simulink model "Latex"  (R2023a)
settings: Solver=VariableStepAuto  StartTime=0.0  StopTime=10.0  RelTol=1e-3
undefined symbols (not defined in the file): A, A_motor, B, B_mag0, B_motor, C_motor, D_motor, I, J, K3_2, K_gamma, Ke, Kt, La, n_cal, R_mgt, Ra, RW_omega_max, T_ext, T_max, T_max_mgt
libraries: matrix_library x5, slpidlib x2, vrlib x1
settings Model: Creator=Personal  LastModifiedBy=Personal

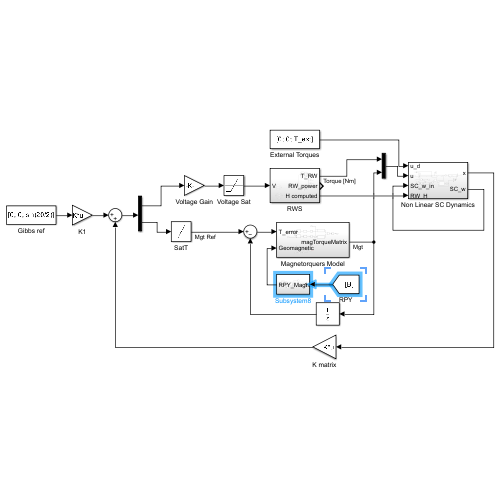
[thumbnail: Simulink's stored preview of the top-level diagram]
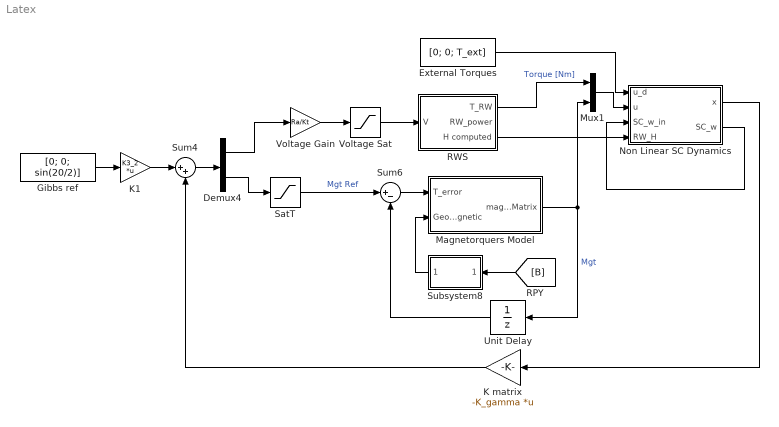
== system Latex ==
  Demux4 : Demux  Outputs=2
  External Torques : Constant  Value=[0; 0; T_ext]
  Gibbs ref : Constant  Value=[0; 0; sin(20/2)]
  K matrix : Gain  Gain=-K_gamma  Multiplication=Matrix(K*u)
  K1 : Gain  Gain=K3_2  Multiplication=Matrix(K*u)
  Magnetorquers Model : Subsystem
  Mux1 : Mux  Inputs=2
  Non Linear SC Dynamics : Subsystem
  RWS : Subsystem
  SatT : Saturate  UpperLimit=T_max_mgt  LowerLimit=-T_max_mgt
  Subsystem8 : Subsystem
  Sum4 : Sum  Inputs=|++
  Sum6 : Sum  Inputs=|+-
  Unit Delay : UnitDelay  SampleTime=-1  HasFrameUpgradeWarning=on
  Voltage Gain : Gain  Gain=Ra/Kt
  Voltage Sat : Saturate  UpperLimit=6  LowerLimit=-6
  wires:
  RWS/3(H computed) -> Non Linear SC Dynamics/4(RW_H)
  Magnetorquers Model/1(magTorqueMatrix) -> Mux1/2, Unit Delay/1  "Mgt"
  SatT/1 -> Sum6/1  "Mgt Ref"
  Non Linear SC Dynamics/2(SC_w) -> Non Linear SC Dynamics/3(SC_w_in)
  [B] -> Subsystem8/1(Input)
  K matrix/1 -> Sum4/2
  Demux4/2 -> SatT/1
  Demux4/1 -> Voltage Gain/1
  Voltage Gain/1 -> Voltage Sat/1
  Sum6/1 -> Magnetorquers Model/1(T_error)
  External Torques/1 -> Non Linear SC Dynamics/1(u_d)
  Voltage Sat/1 -> RWS/1(V)
  K1/1 -> Sum4/1
  Non Linear SC Dynamics/1(x) -> K matrix/1
  RWS/1(T_RW) -> Mux1/1  "Torque [Nm]"
  Mux1/1 -> Non Linear SC Dynamics/2(u)
  Unit Delay/1 -> Sum6/2
  Sum4/1 -> Demux4/1
  Subsystem8/1(RPY_Magnetic) -> Magnetorquers Model/2(Geomagnetic)
  Gibbs ref/1 -> K1/1

== system Latex/Magnetorquers Model ==
  T_error : Inport
  Geomagnetic : Inport  Port=2
  Add : Sum
  Add2 : Sum  Commented=on
  Corrección X : MATLAB Function  TreatAsAtomicUnit=on
  Corrección Y : MATLAB Function  TreatAsAtomicUnit=on
  Demux : Demux  Outputs=3
  From : From  Commented=on  GotoTag=V1
  From1 : From  Commented=on  GotoTag=V2
  Gain : Gain  Commented=on  Gain=1/R_mgt
  Gain1 : Gain  Commented=on  Gain=1/R_mgt
  Geomagnetic1 : InportShadow  Port=2
  Mgt X : Subsystem
  Mgt Y : Subsystem
  PID Controller1 : slpidlib/PID Controller  Controller=PID  Form=Parallel  TimeDomain=Continuous-time  UseExternalTs=off  SampleTime=-1  IntegratorMethod=Forward Euler  FilterMethod=Forward Euler  ControllerParametersSource=internal  P=0  I=2538362.26384975  UseKiTs=off  D=0  N=100  UseFilter=on  TunerSelectOption=Transfer Function Based (PID Tuner App)  InitialConditionSource=internal  InitialConditionForIntegrator=0  InitialConditionForFilter=0  DifferentiatorICPrevScaledInput=0  ExternalReset=none  TrackingMode=off  Kt=1  LimitOutput=on  SatLimitsSource=internal  UpperSaturationLimit=5  LowerSaturationLimit=-5  LinearizeAsGain=on  AntiWindupMode=clamping  Kb=1  LimitIntegrator=off  UpperIntegratorSaturationLimit=inf  LowerIntegratorSaturationLimit=-inf  POutMin=[]  POutMax=[]  IOutMin=[]  IOutMax=[]  DOutMin=[]  DOutMax=[]  NOutMin=[]  NOutMax=[]  SumOutMin=[]  SumOutMax=[]  SaturationOutMin=[]  SaturationOutMax=[]  PParamMin=[]  PParamMax=[]  IParamMin=[]  IParamMax=[]  DParamMin=[]  DParamMax=[]  NParamMin=[]  NParamMax=[]  KbParamMin=[]  KbParamMax=[]  KtParamMin=[]  KtParamMax=[]  KbOutMin=[]  KbOutMax=[]  KtOutMin=[]  KtOutMax=[]  IntegratorOutMin=[]  IntegratorOutMax=[]  FilterOutMin=[]  FilterOutMax=[]  SumI1OutMin=[]  SumI1OutMax=[]  SumI2OutMin=[]  SumI2OutMax=[]  SumI3OutMin=[]  SumI3OutMax=[]  SumI4OutMin=[]  SumI4OutMax=[]  SumDOutMin=[]  SumDOutMax=[]  DifferentiatorOutMin=[]  DifferentiatorOutMax=[]  FilterDiffOutCoefMin=[]  FilterDiffOutCoefMax=[]  ReciprocalOutMin=[]  ReciprocalOutMax=[]  SumDenOutMin=[]  SumDenOutMax=[]  SumNumOutMin=[]  SumNumOutMax=[]  DivideOutMin=[]  DivideOutMax=[]  UdiffTsProdOutMin=[]  UdiffTsProdOutMax=[]  NTsProdOutMin=[]  NTsProdOutMax=[]  UintegralTsProdOutMin=[]  UintegralTsProdOutMax=[]  UngainTsProdOutMin=[]  UngainTsProdOutMax=[]  ClampingZeroOutDataTypeStr=Inherit: Inherit via back propagation  ClampingZeroOutMin=[]  ClampingZeroOutMax=[]  FilterDenConstantOutDataTypeStr=Inherit: Inherit via back propagation  FilterDenConstantOutMin=[]  FilterDenConstantOutMax=[]  PCopyOutDataTypeStr=Inherit: Inherit via back propagation  PCopyOutMin=[]  PCopyOutMax=[]  NCopyOutDataTypeStr=Inherit: Inherit via back propagation  NCopyOutMin=[]  NCopyOutMax=[]  IntegratorContinuousStateAttributes=''  IntegratorStateMustResolveToSignalObject=off  IntegratorRTWStateStorageClass=Auto  FilterContinuousStateAttributes=''  FilterStateMustResolveToSignalObject=off  FilterRTWStateStorageClass=Auto  ParallelPVariant=InternalParameters  IdealPVariant=Disabled  IVariant=InternalParameters  DVariant=InternalParameters  IntegratorVariant=Continuous  SatVariant=Enabled  AWVariant=ContClampingParallel  PCopyVariant=Disabled  TRVariant=Disabled  FdbkBlocksVariant=Forward  IdealPFdbkVariant=Disabled  SatFdbkVariant=Disabled  DerivativeFilterVariant=ContFilter  NVariant=InternalParameters  NCopyVariant=Disabled  FilterICVariant=InternalICsFilter  IntegratorICVariant=InternalICs  ExternalResetVariant=Disabled  TRSumVariant=Passthrough  SumFdbkVariant=Disabled  SumVariant=Sum_PID  TsampFilterVariant=InternalTs  TsampNgainVariant=Passthrough  TsampIntegralVariant=Disabled_SignalSpec  ExternalSaturationOutDataTypeStr=Inherit: Same as second input
  PID Controller5 : slpidlib/PID Controller  Controller=PID  Form=Parallel  TimeDomain=Continuous-time  UseExternalTs=off  SampleTime=-1  IntegratorMethod=Forward Euler  FilterMethod=Forward Euler  ControllerParametersSource=internal  P=0  I=2538362.26384975  UseKiTs=off  D=0  N=100  UseFilter=on  TunerSelectOption=Transfer Function Based (PID Tuner App)  InitialConditionSource=internal  InitialConditionForIntegrator=0  InitialConditionForFilter=0  DifferentiatorICPrevScaledInput=0  ExternalReset=none  TrackingMode=off  Kt=1  LimitOutput=on  SatLimitsSource=internal  UpperSaturationLimit=5  LowerSaturationLimit=-5  LinearizeAsGain=on  AntiWindupMode=clamping  Kb=1  LimitIntegrator=off  UpperIntegratorSaturationLimit=inf  LowerIntegratorSaturationLimit=-inf  POutMin=[]  POutMax=[]  IOutMin=[]  IOutMax=[]  DOutMin=[]  DOutMax=[]  NOutMin=[]  NOutMax=[]  SumOutMin=[]  SumOutMax=[]  SaturationOutMin=[]  SaturationOutMax=[]  PParamMin=[]  PParamMax=[]  IParamMin=[]  IParamMax=[]  DParamMin=[]  DParamMax=[]  NParamMin=[]  NParamMax=[]  KbParamMin=[]  KbParamMax=[]  KtParamMin=[]  KtParamMax=[]  KbOutMin=[]  KbOutMax=[]  KtOutMin=[]  KtOutMax=[]  IntegratorOutMin=[]  IntegratorOutMax=[]  FilterOutMin=[]  FilterOutMax=[]  SumI1OutMin=[]  SumI1OutMax=[]  SumI2OutMin=[]  SumI2OutMax=[]  SumI3OutMin=[]  SumI3OutMax=[]  SumI4OutMin=[]  SumI4OutMax=[]  SumDOutMin=[]  SumDOutMax=[]  DifferentiatorOutMin=[]  DifferentiatorOutMax=[]  FilterDiffOutCoefMin=[]  FilterDiffOutCoefMax=[]  ReciprocalOutMin=[]  ReciprocalOutMax=[]  SumDenOutMin=[]  SumDenOutMax=[]  SumNumOutMin=[]  SumNumOutMax=[]  DivideOutMin=[]  DivideOutMax=[]  UdiffTsProdOutMin=[]  UdiffTsProdOutMax=[]  NTsProdOutMin=[]  NTsProdOutMax=[]  UintegralTsProdOutMin=[]  UintegralTsProdOutMax=[]  UngainTsProdOutMin=[]  UngainTsProdOutMax=[]  ClampingZeroOutDataTypeStr=Inherit: Inherit via back propagation  ClampingZeroOutMin=[]  ClampingZeroOutMax=[]  FilterDenConstantOutDataTypeStr=Inherit: Inherit via back propagation  FilterDenConstantOutMin=[]  FilterDenConstantOutMax=[]  PCopyOutDataTypeStr=Inherit: Inherit via back propagation  PCopyOutMin=[]  PCopyOutMax=[]  NCopyOutDataTypeStr=Inherit: Inherit via back propagation  NCopyOutMin=[]  NCopyOutMax=[]  IntegratorContinuousStateAttributes=''  IntegratorStateMustResolveToSignalObject=off  IntegratorRTWStateStorageClass=Auto  FilterContinuousStateAttributes=''  FilterStateMustResolveToSignalObject=off  FilterRTWStateStorageClass=Auto  ParallelPVariant=InternalParameters  IdealPVariant=Disabled  IVariant=InternalParameters  DVariant=InternalParameters  IntegratorVariant=Continuous  SatVariant=Enabled  AWVariant=ContClampingParallel  PCopyVariant=Disabled  TRVariant=Disabled  FdbkBlocksVariant=Forward  IdealPFdbkVariant=Disabled  SatFdbkVariant=Disabled  DerivativeFilterVariant=ContFilter  NVariant=InternalParameters  NCopyVariant=Disabled  FilterICVariant=InternalICsFilter  IntegratorICVariant=InternalICs  ExternalResetVariant=Disabled  TRSumVariant=Passthrough  SumFdbkVariant=Disabled  SumVariant=Sum_PID  TsampFilterVariant=InternalTs  TsampNgainVariant=Passthrough  TsampIntegralVariant=Disabled_SignalSpec  ExternalSaturationOutDataTypeStr=Inherit: Same as second input
  SatT3 : Saturate  UpperLimit=T_max_mgt  LowerLimit=-T_max_mgt
  Saturation 6V1 : Saturate  UpperLimit=5  LowerLimit=-5
  Saturation 6V2 : Saturate  UpperLimit=5  LowerLimit=-5
  Square : Math  Commented=on  Operator=square
  Square1 : Math  Commented=on  Operator=square
  magTorqueMatrix : Outport
  wires:
  Saturation 6V1/1 -> Mgt X/2(PWR)  "PWR_mgt X"
  PID Controller1/1 -> Saturation 6V2/1
  PID Controller5/1 -> Saturation 6V1/1
  Saturation 6V2/1 -> Mgt Y/2(PWR)  "PWR_mgt Y"
  Add/1 -> SatT3/1
  T_error/1 -> Demux/1
  Mgt X/1(Mgt XYZ) -> Add/1
  Mgt Y/1(Mgt XYZ) -> Add/2
  Demux/3 -> Corrección X/1("T_error "), Corrección Y/1("T_error ")
  Corrección X/1(T_error) -> PID Controller5/1
  Geomagnetic1/1 -> Corrección X/2(B), Corrección Y/2(B)
  Corrección Y/1(T_error) -> PID Controller1/1
  Square1/1 -> Gain1/1
  From/1 -> Square/1
  Gain1/1 -> Add2/2
  Square/1 -> Gain/1
  Gain/1 -> Add2/1
  Add2/1 -> ?
  From1/1 -> Square1/1
  Geomagnetic/1 -> Mgt Y/1(B), Mgt X/1(B)
  SatT3/1 -> magTorqueMatrix/1  "Mgt"

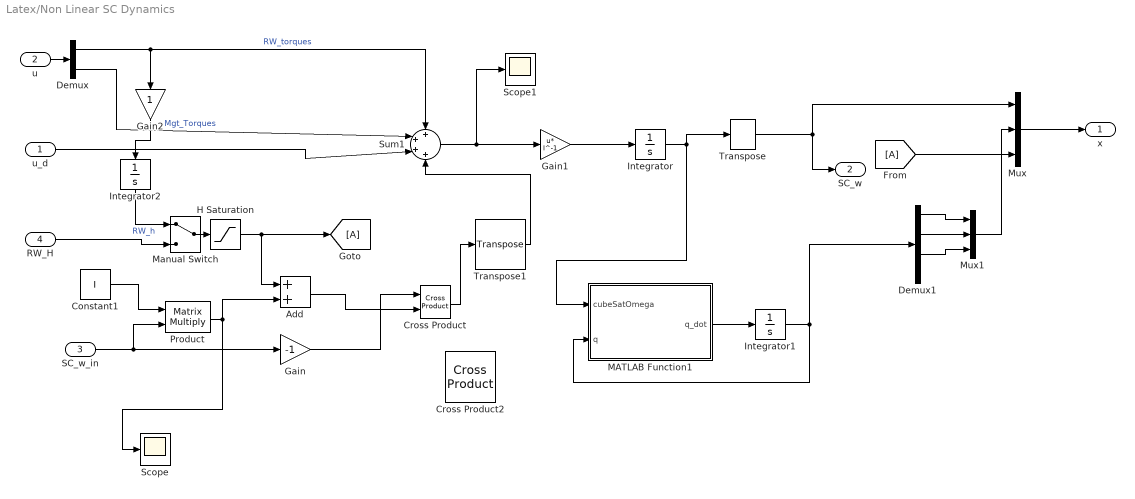
== system Latex/Non Linear SC Dynamics ==
  u_d : Inport
  u : Inport  Port=2
  SC_w_in : Inport  Port=3
  RW_H : Inport  Port=4
  Add : Sum
  Constant1 : Constant  Value=I
  Cross Product : vrlib/Utilities/Cross Product
  Cross Product2 : matrix_library/Cross Product
  Demux : Demux  Outputs=2
  Demux1 : Demux
  From : From
  Gain : Gain  Gain=-1
  Gain1 : Gain  Gain=I^-1  Multiplication=Matrix(u*K)
  Gain2 : Gain
  Goto : Goto
  H Saturation : Saturate  UpperLimit=J*RW_omega_max  LowerLimit=-J*RW_omega_max
  Integrator : Integrator  InitialCondition=[0 0 0]
  Integrator1 : Integrator  InitialCondition=[0 0 0 1]
  Integrator2 : Integrator  InitialCondition=[0 0 0]
  MATLAB Function1 : MATLAB Function  TreatAsAtomicUnit=on
  Manual Switch : ManualSwitch
  Mux : Mux  Inputs=3
  Mux1 : Mux  Inputs=3
  Product : Product  Multiplication=Matrix(*)
  Scope : Scope
  Scope1 : Scope
  Sum1 : Sum  Inputs=++++
  Transpose : matrix_library/Transpose
  Transpose1 : matrix_library/Transpose
  x : Outport
  SC_w : Outport  Port=2
  wires:
  Demux/1 -> Sum1/1, Gain2/1  "RW_torques"
  u_d/1 -> Sum1/3
  Integrator1/1 -> Demux1/1, MATLAB Function1/2(q)
  Constant1/1 -> Product/1
  Product/1 -> Scope/1, Add/2
  Gain/1 -> Cross Product/1
  Add/1 -> Cross Product/2
  Cross Product/1 -> Transpose1/1
  Sum1/1 -> Scope1/1, Gain1/1
  Gain1/1 -> Integrator/1
  Integrator/1 -> MATLAB Function1/1(cubeSatOmega), Transpose/1
  MATLAB Function1/1(q_dot) -> Integrator1/1
  SC_w_in/1 -> Product/2, Gain/1
  Transpose/1 -> SC_w/1, Mux/1
  Transpose1/1 -> Sum1/4
  Demux/2 -> Sum1/2  "Mgt_Torques"
  u/1 -> Demux/1
  Mux/1 -> x/1
  Demux1/1 -> Mux1/1
  Demux1/2 -> Mux1/2
  Demux1/3 -> Mux1/3
  Mux1/1 -> Mux/2
  From/1 -> Mux/3
  H Saturation/1 -> Goto/1, Add/1
  RW_H/1 -> Manual Switch/2
  Manual Switch/1 -> H Saturation/1
  Integrator2/1 -> Manual Switch/1  "RW_h"
  Gain2/1 -> Integrator2/1

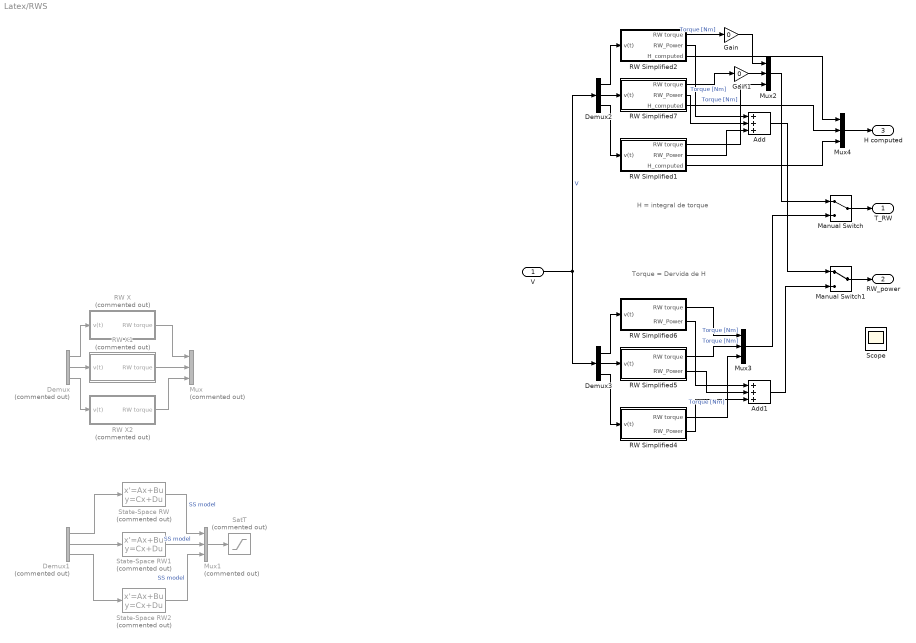
== system Latex/RWS ==
  note: Torque = Dervida de H
  note: H = integral de torque
  V : Inport
  Add : Sum  Inputs=+++
  Add1 : Sum  Inputs=+++
  Demux : Demux  Commented=on  Outputs=3
  Demux1 : Demux  Commented=on  Outputs=3
  Demux2 : Demux  Outputs=3
  Demux3 : Demux  Outputs=3
  Gain : Gain  Gain=0
  Gain1 : Gain  Gain=0
  Manual Switch : ManualSwitch
  Manual Switch1 : ManualSwitch
  Mux : Mux  Commented=on  Inputs=3
  Mux1 : Mux  Commented=on  Inputs=3
  Mux2 : Mux  Inputs=3
  Mux3 : Mux  Inputs=3
  Mux4 : Mux  Inputs=3
  RW Simplified1 : Subsystem
  RW Simplified2 : Subsystem
  RW Simplified4 : Subsystem
  RW Simplified5 : Subsystem
  RW Simplified6 : Subsystem
  RW Simplified7 : Subsystem
  RW X : Subsystem  Commented=on
  RW X1 : Subsystem  Commented=on
  RW X2 : Subsystem  Commented=on
  SatT : Saturate  Commented=on  UpperLimit=T_max  LowerLimit=-T_max
  Scope : Scope
  State-Space RW : StateSpace  Commented=on  A=A_motor  B=B_motor  C=C_motor  D=D_motor  InitialCondition=0
  State-Space RW1 : StateSpace  Commented=on  A=A_motor  B=B_motor  C=C_motor  D=D_motor  InitialCondition=0
  State-Space RW2 : StateSpace  Commented=on  A=A_motor  B=B_motor  C=C_motor  D=D_motor  InitialCondition=0
  T_RW : Outport
  RW_power : Outport  Port=2
  H computed : Outport  Port=3
  wires:
  Demux/1 -> RW X/1(v(t))
  V/1 -> Demux2/1, Demux3/1  "V"
  Demux/3 -> RW X2/1(v(t))
  Demux/2 -> RW X1/1(v(t))
  RW X2/1(RW torque) -> Mux/3
  Demux1/1 -> State-Space RW/1
  Demux1/2 -> State-Space RW1/1
  Demux1/3 -> State-Space RW2/1
  State-Space RW1/1 -> Mux1/2  "SS model"
  State-Space RW/1 -> Mux1/1  "SS model"
  State-Space RW2/1 -> Mux1/3  "SS model"
  Mux1/1 -> SatT/1
  RW Simplified1/2(RW_Power) -> Add/3
  Manual Switch/1 -> T_RW/1
  RW X/1(RW torque) -> Mux/1
  RW X1/1(RW torque) -> Mux/2
  Demux2/1 -> RW Simplified2/1(v(t))
  Demux2/2 -> RW Simplified7/1(v(t))
  Demux2/3 -> RW Simplified1/1(v(t))
  RW Simplified2/1(RW torque) -> Gain/1  "Torque [Nm]"
  RW Simplified7/1(RW torque) -> Gain1/1  "Torque [Nm]"
  RW Simplified1/1(RW torque) -> Mux2/3  "Torque [Nm]"
  Mux2/1 -> Manual Switch/1
  RW Simplified7/2(RW_Power) -> Add/2
  RW Simplified2/2(RW_Power) -> Add/1
  Add/1 -> Manual Switch1/1
  RW Simplified6/2(RW_Power) -> Add1/1
  RW Simplified5/2(RW_Power) -> Add1/2
  Mux3/1 -> Manual Switch/2
  RW Simplified4/1(RW torque) -> Mux3/3  "Torque [Nm]"
  RW Simplified5/1(RW torque) -> Mux3/2  "Torque [Nm]"
  RW Simplified6/1(RW torque) -> Mux3/1  "Torque [Nm]"
  Demux3/3 -> RW Simplified4/1(v(t))
  Demux3/2 -> RW Simplified5/1(v(t))
  Demux3/1 -> RW Simplified6/1(v(t))
  RW Simplified4/2(RW_Power) -> Add1/3
  Add1/1 -> Manual Switch1/2
  Manual Switch1/1 -> RW_power/1
  RW Simplified1/3(H_computed) -> Mux4/3
  RW Simplified2/3(H_computed) -> Mux4/1
  RW Simplified7/3(H_computed) -> Mux4/2
  Mux4/1 -> H computed/1
  Gain/1 -> Mux2/1
  Gain1/1 -> Mux2/2

== system Latex/Subsystem8 ==
  Input : Inport
  Clock : Clock
  Constant1 : Constant  Value=B_mag0
  Extract B : MATLAB Function  TreatAsAtomicUnit=on
  MATLAB Function : MATLAB Function  TreatAsAtomicUnit=on
  Scope1 : Scope
  Scope8 : Scope
  Zero-Order Hold : ZeroOrderHold  SampleTime=-1
  RPY_Magnetic : Outport
  wires:
  Constant1/1 -> Extract B/1(B_cal)
  Extract B/1(XYZ_Magnetic) -> MATLAB Function/1(NEDMagnetic), Scope8/1
  Input/1 -> MATLAB Function/2(RPY)
  Zero-Order Hold/1 -> Scope1/1, Extract B/2(time)
  MATLAB Function/1(RPY_Magnetic) -> RPY_Magnetic/1
  Clock/1 -> Zero-Order Hold/1

== system Latex/Magnetorquers Model/Mgt X ==
  B : Inport
  PWR : Inport  Port=2
  Cross Product : matrix_library/Cross Product
  Mgt_ejeX : Gain  Gain=[1 0 0]
  "Momento Dipolar " : Gain  Gain=n_cal*A/R_mgt
  Mgt XYZ : Outport
  wires:
  "Momento Dipolar "/1 -> Mgt_ejeX/1
  Mgt_ejeX/1 -> Cross Product/1
  Cross Product/1 -> Mgt XYZ/1  "MgtX"
  PWR/1 -> "Momento Dipolar "/1
  B/1 -> Cross Product/2

== system Latex/Magnetorquers Model/Mgt Y ==
  B : Inport
  PWR : Inport  Port=2
  Cross Product : matrix_library/Cross Product
  Mgt_ejeY : Gain  Gain=[0 1 0]
  "Momento Dipolar " : Gain  Gain=n_cal*A/R_mgt
  Mgt XYZ : Outport
  wires:
  B/1 -> Cross Product/2
  PWR/1 -> "Momento Dipolar "/1
  Cross Product/1 -> Mgt XYZ/1  "MgtX"
  Mgt_ejeY/1 -> Cross Product/1
  "Momento Dipolar "/1 -> Mgt_ejeY/1

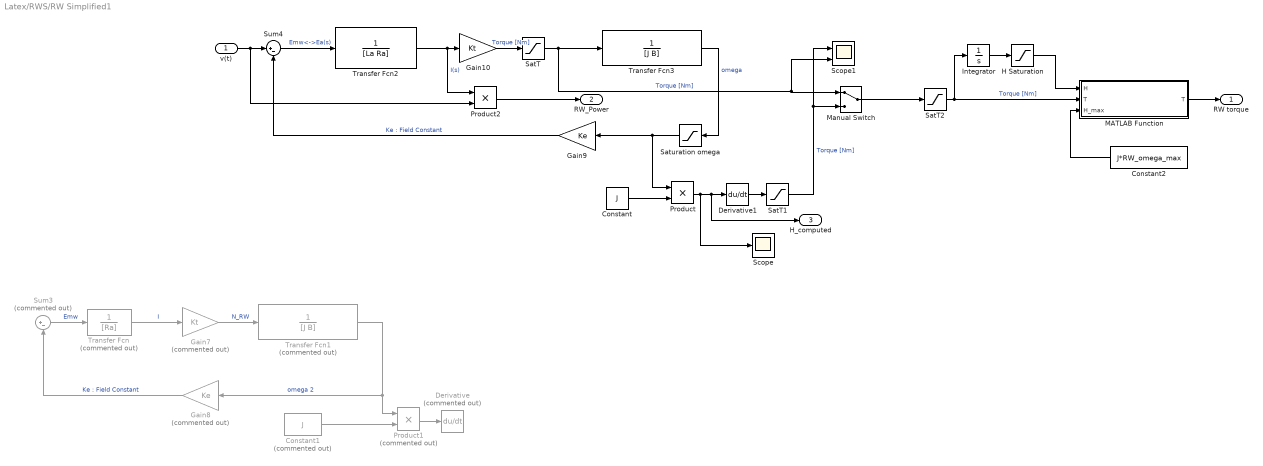
== system Latex/RWS/RW Simplified1 ==
  v(t) : Inport
  Constant : Constant  Value=J
  Constant1 : Constant  Commented=on  Value=J
  Constant2 : Constant  Value=J*RW_omega_max
  Derivative : Derivative  Commented=on
  Derivative1 : Derivative
  Gain10 : Gain  Gain=Kt
  Gain7 : Gain  Commented=on  Gain=Kt
  Gain8 : Gain  Commented=on  Gain=Ke
  Gain9 : Gain  Gain=Ke
  H Saturation : Saturate  UpperLimit=J*RW_omega_max  LowerLimit=-J*RW_omega_max
  Integrator : Integrator
  MATLAB Function : MATLAB Function  TreatAsAtomicUnit=on
  Manual Switch : ManualSwitch
  Product : Product
  Product1 : Product  Commented=on
  Product2 : Product
  SatT : Saturate  UpperLimit=T_max  LowerLimit=-T_max
  SatT1 : Saturate  UpperLimit=T_max  LowerLimit=-T_max
  SatT2 : Saturate  UpperLimit=T_max  LowerLimit=-T_max
  Saturation omega : Saturate  UpperLimit=RW_omega_max  LowerLimit=-RW_omega_max
  Scope : Scope
  Scope1 : Scope  NumInputPorts=2
  Sum3 : Sum  Commented=on  Inputs=|+-
  Sum4 : Sum  Inputs=|+-
  Transfer Fcn : TransferFcn  Commented=on  Denominator=[Ra]
  Transfer Fcn1 : TransferFcn  Commented=on  Denominator=[J B]
  Transfer Fcn2 : TransferFcn  Denominator=[La Ra]
  Transfer Fcn3 : TransferFcn  Denominator=[J B]
  RW torque : Outport  VectorParamsAs1DForOutWhenUnconnected=off
  RW_Power : Outport  Port=2  VectorParamsAs1DForOutWhenUnconnected=off
  H_computed : Outport  Port=3
  wires:
  Transfer Fcn2/1 -> Product2/1, Gain10/1  "I(s)"
  Sum4/1 -> Transfer Fcn2/1  "Emw<->Ea(s)"
  Gain9/1 -> Sum4/2  "Ke : Field Constant"
  Transfer Fcn3/1 -> Saturation omega/1  "omega"
  Constant/1 -> Product/2
  v(t)/1 -> Product2/2, Sum4/1
  Product1/1 -> Derivative/1
  Constant1/1 -> Product1/2
  Transfer Fcn1/1 -> Product1/1, Gain8/1  "omega 2"
  Gain7/1 -> Transfer Fcn1/1  "N_RW"
  Sum3/1 -> Transfer Fcn/1  "Emw"
  Transfer Fcn/1 -> Gain7/1  "I"
  Gain8/1 -> Sum3/2  "Ke : Field Constant"
  Gain10/1 -> SatT/1  "Torque [Nm]"
  SatT/1 -> Manual Switch/1, Scope1/2, Transfer Fcn3/1  "Torque [Nm]"
  Product2/1 -> RW_Power/1
  Product/1 -> Scope/1, H_computed/1, Derivative1/1
  Derivative1/1 -> SatT1/1
  SatT1/1 -> Scope1/1, Manual Switch/2  "Torque [Nm]"
  Manual Switch/1 -> SatT2/1
  Saturation omega/1 -> Product/1, Gain9/1
  SatT2/1 -> MATLAB Function/2("T "), Integrator/1  "Torque [Nm]"
  Integrator/1 -> H Saturation/1
  Constant2/1 -> MATLAB Function/3(H_max)
  H Saturation/1 -> MATLAB Function/1(H)
  MATLAB Function/1(T) -> RW torque/1

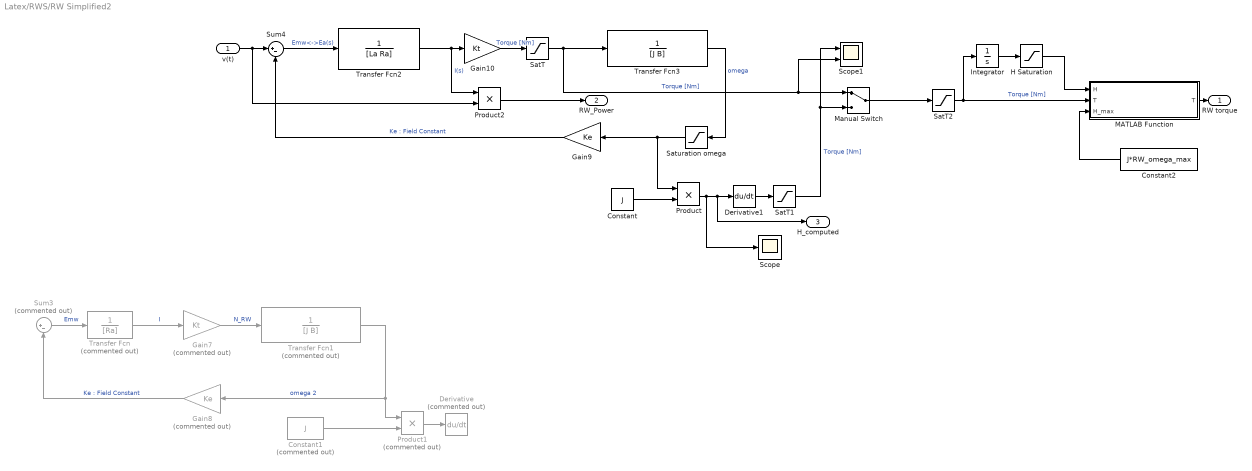
== system Latex/RWS/RW Simplified2 ==
  v(t) : Inport
  Constant : Constant  Value=J
  Constant1 : Constant  Commented=on  Value=J
  Constant2 : Constant  Value=J*RW_omega_max
  Derivative : Derivative  Commented=on
  Derivative1 : Derivative
  Gain10 : Gain  Gain=Kt
  Gain7 : Gain  Commented=on  Gain=Kt
  Gain8 : Gain  Commented=on  Gain=Ke
  Gain9 : Gain  Gain=Ke
  H Saturation : Saturate  UpperLimit=J*RW_omega_max  LowerLimit=-J*RW_omega_max
  Integrator : Integrator
  MATLAB Function : MATLAB Function  TreatAsAtomicUnit=on
  Manual Switch : ManualSwitch
  Product : Product
  Product1 : Product  Commented=on
  Product2 : Product
  SatT : Saturate  UpperLimit=T_max  LowerLimit=-T_max
  SatT1 : Saturate  UpperLimit=T_max  LowerLimit=-T_max
  SatT2 : Saturate  UpperLimit=T_max  LowerLimit=-T_max
  Saturation omega : Saturate  UpperLimit=RW_omega_max  LowerLimit=-RW_omega_max
  Scope : Scope
  Scope1 : Scope  NumInputPorts=2
  Sum3 : Sum  Commented=on  Inputs=|+-
  Sum4 : Sum  Inputs=|+-
  Transfer Fcn : TransferFcn  Commented=on  Denominator=[Ra]
  Transfer Fcn1 : TransferFcn  Commented=on  Denominator=[J B]
  Transfer Fcn2 : TransferFcn  Denominator=[La Ra]
  Transfer Fcn3 : TransferFcn  Denominator=[J B]
  RW torque : Outport  VectorParamsAs1DForOutWhenUnconnected=off
  RW_Power : Outport  Port=2  VectorParamsAs1DForOutWhenUnconnected=off
  H_computed : Outport  Port=3
  wires:
  Transfer Fcn2/1 -> Product2/1, Gain10/1  "I(s)"
  Sum4/1 -> Transfer Fcn2/1  "Emw<->Ea(s)"
  Gain9/1 -> Sum4/2  "Ke : Field Constant"
  Transfer Fcn3/1 -> Saturation omega/1  "omega"
  Constant/1 -> Product/2
  v(t)/1 -> Product2/2, Sum4/1
  Product1/1 -> Derivative/1
  Constant1/1 -> Product1/2
  Transfer Fcn1/1 -> Product1/1, Gain8/1  "omega 2"
  Gain7/1 -> Transfer Fcn1/1  "N_RW"
  Sum3/1 -> Transfer Fcn/1  "Emw"
  Transfer Fcn/1 -> Gain7/1  "I"
  Gain8/1 -> Sum3/2  "Ke : Field Constant"
  Gain10/1 -> SatT/1  "Torque [Nm]"
  SatT/1 -> Manual Switch/1, Scope1/2, Transfer Fcn3/1  "Torque [Nm]"
  Product2/1 -> RW_Power/1
  Product/1 -> Scope/1, H_computed/1, Derivative1/1
  Derivative1/1 -> SatT1/1
  SatT1/1 -> Scope1/1, Manual Switch/2  "Torque [Nm]"
  Manual Switch/1 -> SatT2/1
  Saturation omega/1 -> Product/1, Gain9/1
  SatT2/1 -> Integrator/1, MATLAB Function/2("T ")  "Torque [Nm]"
  Integrator/1 -> H Saturation/1
  Constant2/1 -> MATLAB Function/3(H_max)
  H Saturation/1 -> MATLAB Function/1(H)
  MATLAB Function/1(T) -> RW torque/1

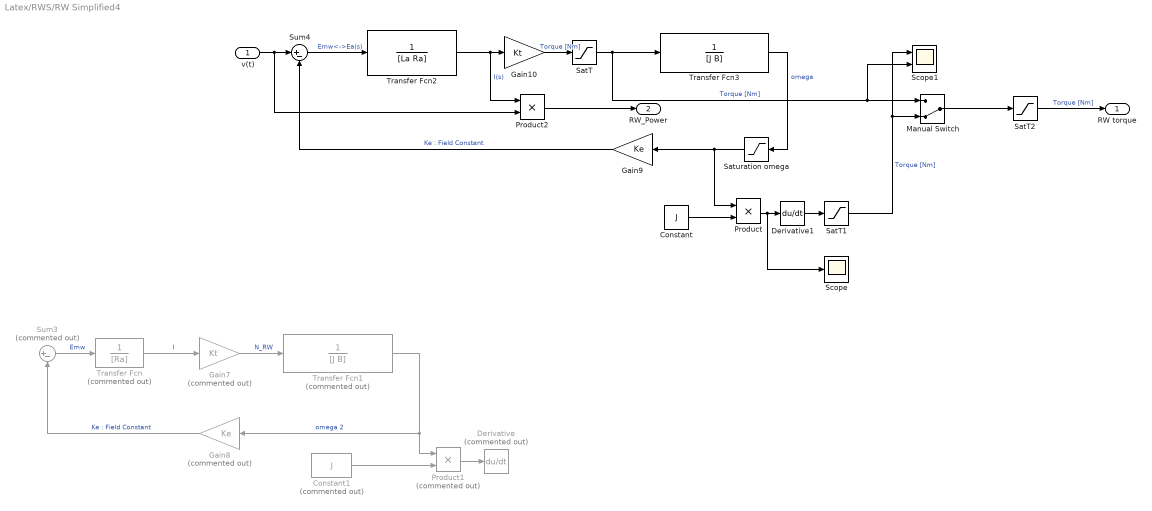
== system Latex/RWS/RW Simplified4 ==
  v(t) : Inport
  Constant : Constant  Value=J
  Constant1 : Constant  Commented=on  Value=J
  Derivative : Derivative  Commented=on
  Derivative1 : Derivative
  Gain10 : Gain  Gain=Kt
  Gain7 : Gain  Commented=on  Gain=Kt
  Gain8 : Gain  Commented=on  Gain=Ke
  Gain9 : Gain  Gain=Ke
  Manual Switch : ManualSwitch  CurrentSetting=0
  Product : Product
  Product1 : Product  Commented=on
  Product2 : Product
  SatT : Saturate  UpperLimit=T_max  LowerLimit=-T_max
  SatT1 : Saturate  UpperLimit=T_max  LowerLimit=-T_max
  SatT2 : Saturate  UpperLimit=T_max  LowerLimit=-T_max
  Saturation omega : Saturate  UpperLimit=RW_omega_max  LowerLimit=-RW_omega_max
  Scope : Scope
  Scope1 : Scope  NumInputPorts=2
  Sum3 : Sum  Commented=on  Inputs=|+-
  Sum4 : Sum  Inputs=|+-
  Transfer Fcn : TransferFcn  Commented=on  Denominator=[Ra]
  Transfer Fcn1 : TransferFcn  Commented=on  Denominator=[J B]
  Transfer Fcn2 : TransferFcn  Denominator=[La Ra]
  Transfer Fcn3 : TransferFcn  Denominator=[J B]
  RW torque : Outport  VectorParamsAs1DForOutWhenUnconnected=off
  RW_Power : Outport  Port=2  VectorParamsAs1DForOutWhenUnconnected=off
  wires:
  SatT2/1 -> RW torque/1  "Torque [Nm]"
  Saturation omega/1 -> Gain9/1, Product/1
  Manual Switch/1 -> SatT2/1
  SatT1/1 -> Manual Switch/2, Scope1/1  "Torque [Nm]"
  Derivative1/1 -> SatT1/1
  Product/1 -> Derivative1/1, Scope/1
  Product2/1 -> RW_Power/1
  SatT/1 -> Transfer Fcn3/1, Scope1/2, Manual Switch/1  "Torque [Nm]"
  Gain10/1 -> SatT/1  "Torque [Nm]"
  Gain8/1 -> Sum3/2  "Ke : Field Constant"
  Transfer Fcn/1 -> Gain7/1  "I"
  Sum3/1 -> Transfer Fcn/1  "Emw"
  Gain7/1 -> Transfer Fcn1/1  "N_RW"
  Transfer Fcn1/1 -> Gain8/1, Product1/1  "omega 2"
  Constant1/1 -> Product1/2
  Product1/1 -> Derivative/1
  v(t)/1 -> Sum4/1, Product2/2
  Constant/1 -> Product/2
  Transfer Fcn3/1 -> Saturation omega/1  "omega"
  Gain9/1 -> Sum4/2  "Ke : Field Constant"
  Sum4/1 -> Transfer Fcn2/1  "Emw<->Ea(s)"
  Transfer Fcn2/1 -> Gain10/1, Product2/1  "I(s)"

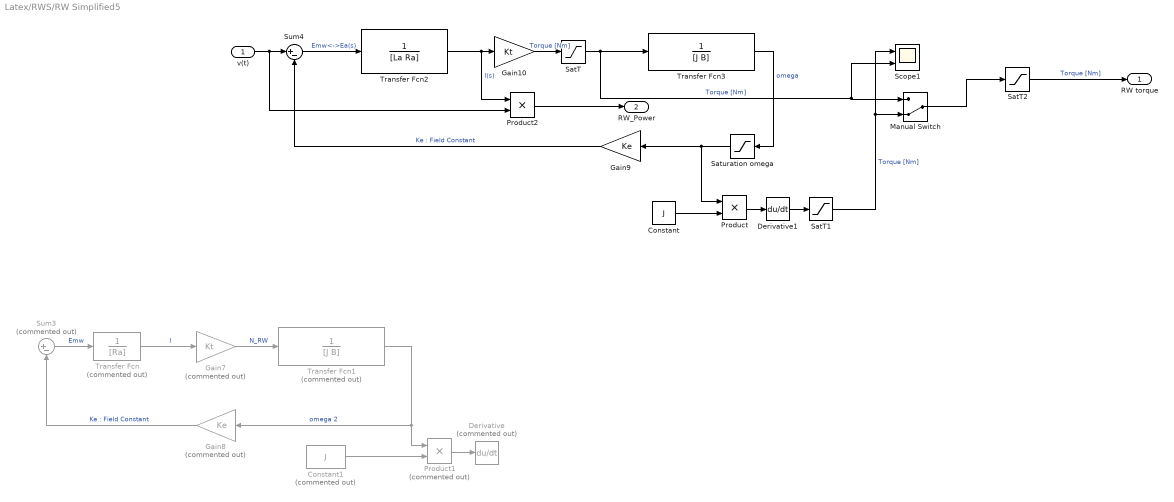
== system Latex/RWS/RW Simplified5 ==
  v(t) : Inport
  Constant : Constant  Value=J
  Constant1 : Constant  Commented=on  Value=J
  Derivative : Derivative  Commented=on
  Derivative1 : Derivative
  Gain10 : Gain  Gain=Kt
  Gain7 : Gain  Commented=on  Gain=Kt
  Gain8 : Gain  Commented=on  Gain=Ke
  Gain9 : Gain  Gain=Ke
  Manual Switch : ManualSwitch  CurrentSetting=0
  Product : Product
  Product1 : Product  Commented=on
  Product2 : Product
  SatT : Saturate  UpperLimit=T_max  LowerLimit=-T_max
  SatT1 : Saturate  UpperLimit=T_max  LowerLimit=-T_max
  SatT2 : Saturate  UpperLimit=T_max  LowerLimit=-T_max
  Saturation omega : Saturate  UpperLimit=RW_omega_max  LowerLimit=-RW_omega_max
  Scope1 : Scope  NumInputPorts=2
  Sum3 : Sum  Commented=on  Inputs=|+-
  Sum4 : Sum  Inputs=|+-
  Transfer Fcn : TransferFcn  Commented=on  Denominator=[Ra]
  Transfer Fcn1 : TransferFcn  Commented=on  Denominator=[J B]
  Transfer Fcn2 : TransferFcn  Denominator=[La Ra]
  Transfer Fcn3 : TransferFcn  Denominator=[J B]
  RW torque : Outport  VectorParamsAs1DForOutWhenUnconnected=off
  RW_Power : Outport  Port=2  VectorParamsAs1DForOutWhenUnconnected=off
  wires:
  Transfer Fcn2/1 -> Product2/1, Gain10/1  "I(s)"
  Sum4/1 -> Transfer Fcn2/1  "Emw<->Ea(s)"
  Gain9/1 -> Sum4/2  "Ke : Field Constant"
  Transfer Fcn3/1 -> Saturation omega/1  "omega"
  Constant/1 -> Product/2
  v(t)/1 -> Product2/2, Sum4/1
  Product1/1 -> Derivative/1
  Constant1/1 -> Product1/2
  Transfer Fcn1/1 -> Product1/1, Gain8/1  "omega 2"
  Gain7/1 -> Transfer Fcn1/1  "N_RW"
  Sum3/1 -> Transfer Fcn/1  "Emw"
  Transfer Fcn/1 -> Gain7/1  "I"
  Gain8/1 -> Sum3/2  "Ke : Field Constant"
  Gain10/1 -> SatT/1  "Torque [Nm]"
  SatT/1 -> Manual Switch/1, Scope1/2, Transfer Fcn3/1  "Torque [Nm]"
  Product2/1 -> RW_Power/1
  Product/1 -> Derivative1/1
  Derivative1/1 -> SatT1/1
  SatT1/1 -> Scope1/1, Manual Switch/2  "Torque [Nm]"
  Manual Switch/1 -> SatT2/1
  Saturation omega/1 -> Product/1, Gain9/1
  SatT2/1 -> RW torque/1  "Torque [Nm]"

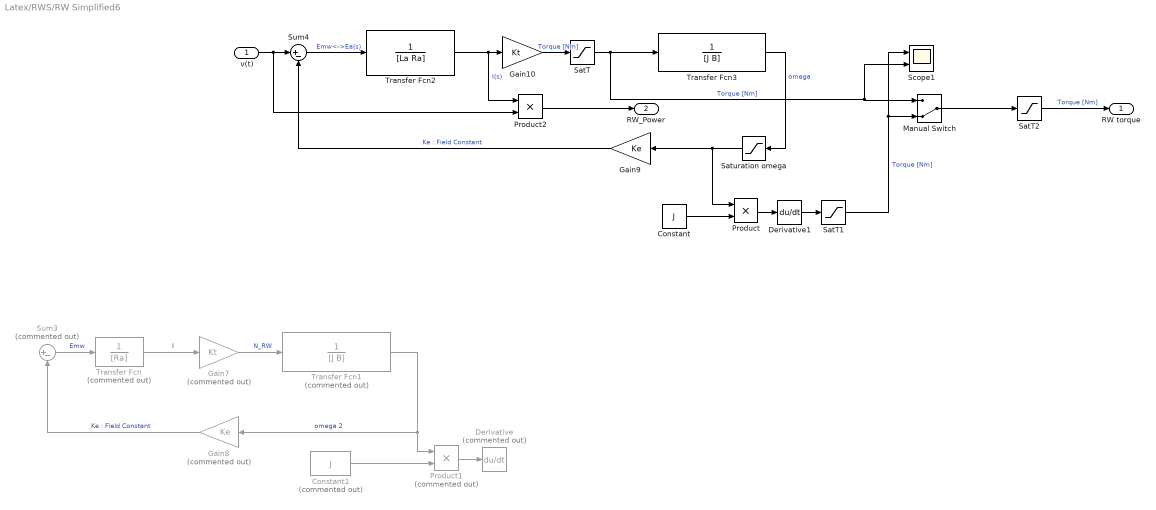
== system Latex/RWS/RW Simplified6 ==
  v(t) : Inport
  Constant : Constant  Value=J
  Constant1 : Constant  Commented=on  Value=J
  Derivative : Derivative  Commented=on
  Derivative1 : Derivative
  Gain10 : Gain  Gain=Kt
  Gain7 : Gain  Commented=on  Gain=Kt
  Gain8 : Gain  Commented=on  Gain=Ke
  Gain9 : Gain  Gain=Ke
  Manual Switch : ManualSwitch  CurrentSetting=0
  Product : Product
  Product1 : Product  Commented=on
  Product2 : Product
  SatT : Saturate  UpperLimit=T_max  LowerLimit=-T_max
  SatT1 : Saturate  UpperLimit=T_max  LowerLimit=-T_max
  SatT2 : Saturate  UpperLimit=T_max  LowerLimit=-T_max
  Saturation omega : Saturate  UpperLimit=RW_omega_max  LowerLimit=-RW_omega_max
  Scope1 : Scope  NumInputPorts=2
  Sum3 : Sum  Commented=on  Inputs=|+-
  Sum4 : Sum  Inputs=|+-
  Transfer Fcn : TransferFcn  Commented=on  Denominator=[Ra]
  Transfer Fcn1 : TransferFcn  Commented=on  Denominator=[J B]
  Transfer Fcn2 : TransferFcn  Denominator=[La Ra]
  Transfer Fcn3 : TransferFcn  Denominator=[J B]
  RW torque : Outport  VectorParamsAs1DForOutWhenUnconnected=off
  RW_Power : Outport  Port=2  VectorParamsAs1DForOutWhenUnconnected=off
  wires:
  SatT2/1 -> RW torque/1  "Torque [Nm]"
  Saturation omega/1 -> Gain9/1, Product/1
  Manual Switch/1 -> SatT2/1
  SatT1/1 -> Manual Switch/2, Scope1/1  "Torque [Nm]"
  Derivative1/1 -> SatT1/1
  Product/1 -> Derivative1/1
  Product2/1 -> RW_Power/1
  SatT/1 -> Transfer Fcn3/1, Scope1/2, Manual Switch/1  "Torque [Nm]"
  Gain10/1 -> SatT/1  "Torque [Nm]"
  Gain8/1 -> Sum3/2  "Ke : Field Constant"
  Transfer Fcn/1 -> Gain7/1  "I"
  Sum3/1 -> Transfer Fcn/1  "Emw"
  Gain7/1 -> Transfer Fcn1/1  "N_RW"
  Transfer Fcn1/1 -> Gain8/1, Product1/1  "omega 2"
  Constant1/1 -> Product1/2
  Product1/1 -> Derivative/1
  v(t)/1 -> Sum4/1, Product2/2
  Constant/1 -> Product/2
  Transfer Fcn3/1 -> Saturation omega/1  "omega"
  Gain9/1 -> Sum4/2  "Ke : Field Constant"
  Sum4/1 -> Transfer Fcn2/1  "Emw<->Ea(s)"
  Transfer Fcn2/1 -> Gain10/1, Product2/1  "I(s)"

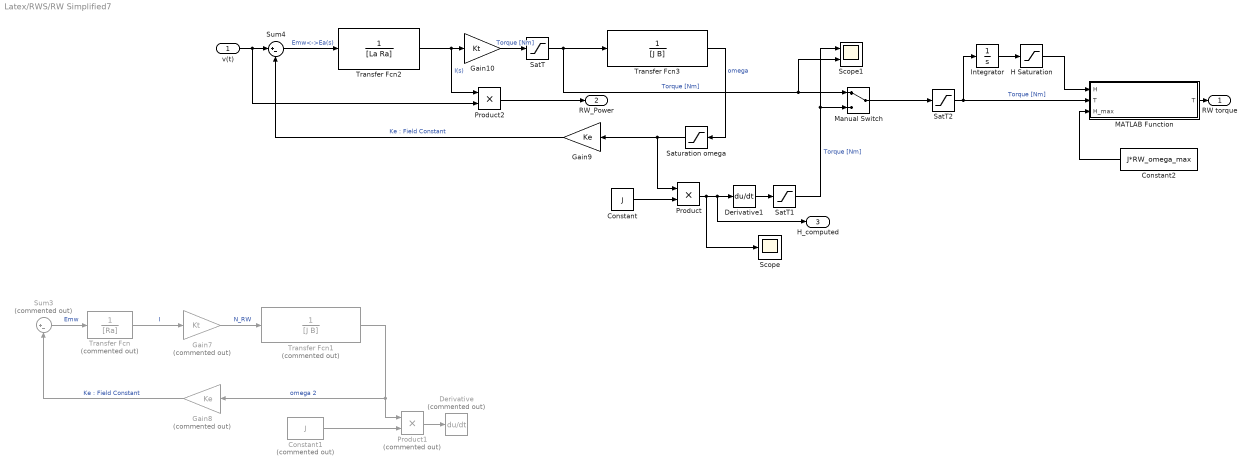
== system Latex/RWS/RW Simplified7 ==
  v(t) : Inport
  Constant : Constant  Value=J
  Constant1 : Constant  Commented=on  Value=J
  Constant2 : Constant  Value=J*RW_omega_max
  Derivative : Derivative  Commented=on
  Derivative1 : Derivative
  Gain10 : Gain  Gain=Kt
  Gain7 : Gain  Commented=on  Gain=Kt
  Gain8 : Gain  Commented=on  Gain=Ke
  Gain9 : Gain  Gain=Ke
  H Saturation : Saturate  UpperLimit=J*RW_omega_max  LowerLimit=-J*RW_omega_max
  Integrator : Integrator
  MATLAB Function : MATLAB Function  TreatAsAtomicUnit=on
  Manual Switch : ManualSwitch
  Product : Product
  Product1 : Product  Commented=on
  Product2 : Product
  SatT : Saturate  UpperLimit=T_max  LowerLimit=-T_max
  SatT1 : Saturate  UpperLimit=T_max  LowerLimit=-T_max
  SatT2 : Saturate  UpperLimit=T_max  LowerLimit=-T_max
  Saturation omega : Saturate  UpperLimit=RW_omega_max  LowerLimit=-RW_omega_max
  Scope : Scope
  Scope1 : Scope  NumInputPorts=2
  Sum3 : Sum  Commented=on  Inputs=|+-
  Sum4 : Sum  Inputs=|+-
  Transfer Fcn : TransferFcn  Commented=on  Denominator=[Ra]
  Transfer Fcn1 : TransferFcn  Commented=on  Denominator=[J B]
  Transfer Fcn2 : TransferFcn  Denominator=[La Ra]
  Transfer Fcn3 : TransferFcn  Denominator=[J B]
  RW torque : Outport  VectorParamsAs1DForOutWhenUnconnected=off
  RW_Power : Outport  Port=2  VectorParamsAs1DForOutWhenUnconnected=off
  H_computed : Outport  Port=3
  wires:
  MATLAB Function/1(T) -> RW torque/1
  H Saturation/1 -> MATLAB Function/1(H)
  Constant2/1 -> MATLAB Function/3(H_max)
  Integrator/1 -> H Saturation/1
  SatT2/1 -> MATLAB Function/2("T "), Integrator/1  "Torque [Nm]"
  Saturation omega/1 -> Gain9/1, Product/1
  Manual Switch/1 -> SatT2/1
  SatT1/1 -> Manual Switch/2, Scope1/1  "Torque [Nm]"
  Derivative1/1 -> SatT1/1
  Product/1 -> Derivative1/1, H_computed/1, Scope/1
  Product2/1 -> RW_Power/1
  SatT/1 -> Transfer Fcn3/1, Scope1/2, Manual Switch/1  "Torque [Nm]"
  Gain10/1 -> SatT/1  "Torque [Nm]"
  Gain8/1 -> Sum3/2  "Ke : Field Constant"
  Transfer Fcn/1 -> Gain7/1  "I"
  Sum3/1 -> Transfer Fcn/1  "Emw"
  Gain7/1 -> Transfer Fcn1/1  "N_RW"
  Transfer Fcn1/1 -> Gain8/1, Product1/1  "omega 2"
  Constant1/1 -> Product1/2
  Product1/1 -> Derivative/1
  v(t)/1 -> Sum4/1, Product2/2
  Constant/1 -> Product/2
  Transfer Fcn3/1 -> Saturation omega/1  "omega"
  Gain9/1 -> Sum4/2  "Ke : Field Constant"
  Sum4/1 -> Transfer Fcn2/1  "Emw<->Ea(s)"
  Transfer Fcn2/1 -> Gain10/1, Product2/1  "I(s)"

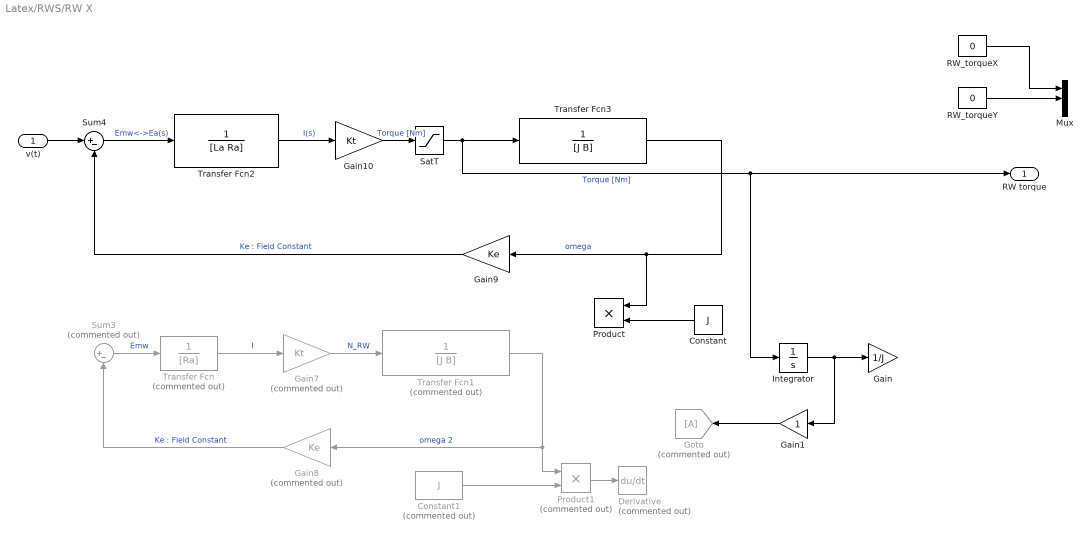
== system Latex/RWS/RW X ==
  v(t) : Inport
  Constant : Constant  Value=J
  Constant1 : Constant  Commented=on  Value=J
  Derivative : Derivative  Commented=on
  Gain : Gain  Gain=1/J
  Gain1 : Gain
  Gain10 : Gain  Gain=Kt
  Gain7 : Gain  Commented=on  Gain=Kt
  Gain8 : Gain  Commented=on  Gain=Ke
  Gain9 : Gain  Gain=Ke
  Goto : Goto  Commented=on
  Integrator : Integrator
  Mux : Mux  Inputs=3
  Product : Product
  Product1 : Product  Commented=on
  RW_torqueX : Constant  Value=0
  RW_torqueY : Constant  Value=0
  SatT : Saturate  UpperLimit=T_max  LowerLimit=-T_max
  Sum3 : Sum  Commented=on  Inputs=|+-
  Sum4 : Sum  Inputs=|+-
  Transfer Fcn : TransferFcn  Commented=on  Denominator=[Ra]
  Transfer Fcn1 : TransferFcn  Commented=on  Denominator=[J B]
  Transfer Fcn2 : TransferFcn  Denominator=[La Ra]
  Transfer Fcn3 : TransferFcn  Denominator=[J B]
  RW torque : Outport  VectorParamsAs1DForOutWhenUnconnected=off
  wires:
  SatT/1 -> Transfer Fcn3/1, Integrator/1, RW torque/1  "Torque [Nm]"
  Gain1/1 -> Goto/1
  Gain10/1 -> SatT/1  "Torque [Nm]"
  RW_torqueY/1 -> Mux/2
  RW_torqueX/1 -> Mux/1
  Gain8/1 -> Sum3/2  "Ke : Field Constant"
  Transfer Fcn/1 -> Gain7/1  "I"
  Sum3/1 -> Transfer Fcn/1  "Emw"
  Gain7/1 -> Transfer Fcn1/1  "N_RW"
  Transfer Fcn1/1 -> Gain8/1, Product1/1  "omega 2"
  Constant1/1 -> Product1/2
  Product1/1 -> Derivative/1
  v(t)/1 -> Sum4/1
  Integrator/1 -> Gain/1, Gain1/1
  Constant/1 -> Product/2
  Transfer Fcn3/1 -> Product/1, Gain9/1  "omega"
  Gain9/1 -> Sum4/2  "Ke : Field Constant"
  Sum4/1 -> Transfer Fcn2/1  "Emw<->Ea(s)"
  Transfer Fcn2/1 -> Gain10/1  "I(s)"

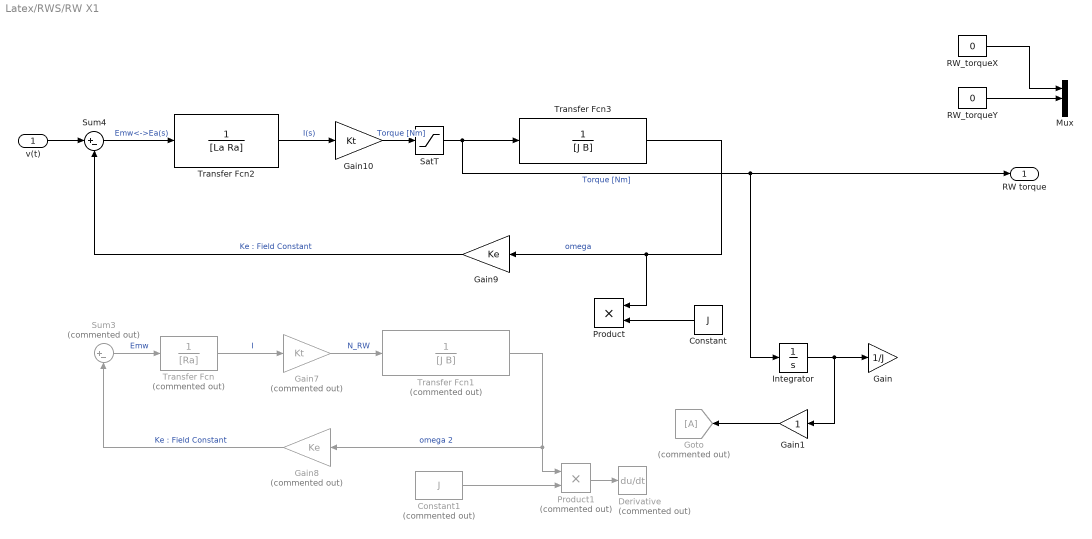
== system Latex/RWS/RW X1 ==
  v(t) : Inport
  Constant : Constant  Value=J
  Constant1 : Constant  Commented=on  Value=J
  Derivative : Derivative  Commented=on
  Gain : Gain  Gain=1/J
  Gain1 : Gain
  Gain10 : Gain  Gain=Kt
  Gain7 : Gain  Commented=on  Gain=Kt
  Gain8 : Gain  Commented=on  Gain=Ke
  Gain9 : Gain  Gain=Ke
  Goto : Goto  Commented=on
  Integrator : Integrator
  Mux : Mux  Inputs=3
  Product : Product
  Product1 : Product  Commented=on
  RW_torqueX : Constant  Value=0
  RW_torqueY : Constant  Value=0
  SatT : Saturate  UpperLimit=T_max  LowerLimit=-T_max
  Sum3 : Sum  Commented=on  Inputs=|+-
  Sum4 : Sum  Inputs=|+-
  Transfer Fcn : TransferFcn  Commented=on  Denominator=[Ra]
  Transfer Fcn1 : TransferFcn  Commented=on  Denominator=[J B]
  Transfer Fcn2 : TransferFcn  Denominator=[La Ra]
  Transfer Fcn3 : TransferFcn  Denominator=[J B]
  RW torque : Outport  VectorParamsAs1DForOutWhenUnconnected=off
  wires:
  Transfer Fcn2/1 -> Gain10/1  "I(s)"
  Sum4/1 -> Transfer Fcn2/1  "Emw<->Ea(s)"
  Gain9/1 -> Sum4/2  "Ke : Field Constant"
  Transfer Fcn3/1 -> Gain9/1, Product/1  "omega"
  Constant/1 -> Product/2
  Integrator/1 -> Gain1/1, Gain/1
  v(t)/1 -> Sum4/1
  Product1/1 -> Derivative/1
  Constant1/1 -> Product1/2
  Transfer Fcn1/1 -> Product1/1, Gain8/1  "omega 2"
  Gain7/1 -> Transfer Fcn1/1  "N_RW"
  Sum3/1 -> Transfer Fcn/1  "Emw"
  Transfer Fcn/1 -> Gain7/1  "I"
  Gain8/1 -> Sum3/2  "Ke : Field Constant"
  RW_torqueX/1 -> Mux/1
  RW_torqueY/1 -> Mux/2
  Gain10/1 -> SatT/1  "Torque [Nm]"
  Gain1/1 -> Goto/1
  SatT/1 -> RW torque/1, Integrator/1, Transfer Fcn3/1  "Torque [Nm]"

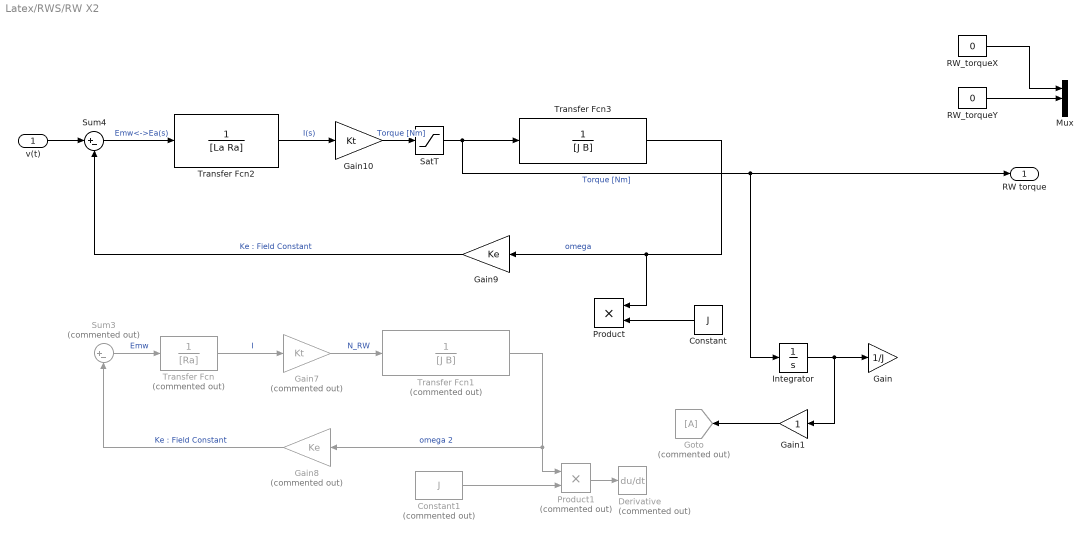
== system Latex/RWS/RW X2 ==
  v(t) : Inport
  Constant : Constant  Value=J
  Constant1 : Constant  Commented=on  Value=J
  Derivative : Derivative  Commented=on
  Gain : Gain  Gain=1/J
  Gain1 : Gain
  Gain10 : Gain  Gain=Kt
  Gain7 : Gain  Commented=on  Gain=Kt
  Gain8 : Gain  Commented=on  Gain=Ke
  Gain9 : Gain  Gain=Ke
  Goto : Goto  Commented=on
  Integrator : Integrator
  Mux : Mux  Inputs=3
  Product : Product
  Product1 : Product  Commented=on
  RW_torqueX : Constant  Value=0
  RW_torqueY : Constant  Value=0
  SatT : Saturate  UpperLimit=T_max  LowerLimit=-T_max
  Sum3 : Sum  Commented=on  Inputs=|+-
  Sum4 : Sum  Inputs=|+-
  Transfer Fcn : TransferFcn  Commented=on  Denominator=[Ra]
  Transfer Fcn1 : TransferFcn  Commented=on  Denominator=[J B]
  Transfer Fcn2 : TransferFcn  Denominator=[La Ra]
  Transfer Fcn3 : TransferFcn  Denominator=[J B]
  RW torque : Outport  VectorParamsAs1DForOutWhenUnconnected=off
  wires:
  SatT/1 -> Transfer Fcn3/1, Integrator/1, RW torque/1  "Torque [Nm]"
  Gain1/1 -> Goto/1
  Gain10/1 -> SatT/1  "Torque [Nm]"
  RW_torqueY/1 -> Mux/2
  RW_torqueX/1 -> Mux/1
  Gain8/1 -> Sum3/2  "Ke : Field Constant"
  Transfer Fcn/1 -> Gain7/1  "I"
  Sum3/1 -> Transfer Fcn/1  "Emw"
  Gain7/1 -> Transfer Fcn1/1  "N_RW"
  Transfer Fcn1/1 -> Gain8/1, Product1/1  "omega 2"
  Constant1/1 -> Product1/2
  Product1/1 -> Derivative/1
  v(t)/1 -> Sum4/1
  Integrator/1 -> Gain/1, Gain1/1
  Constant/1 -> Product/2
  Transfer Fcn3/1 -> Product/1, Gain9/1  "omega"
  Gain9/1 -> Sum4/2  "Ke : Field Constant"
  Sum4/1 -> Transfer Fcn2/1  "Emw<->Ea(s)"
  Transfer Fcn2/1 -> Gain10/1  "I(s)"

== matlab function Latex/RWS/RW Simplified1/MATLAB Function ==
  data: H input; T output; T input; H_max input
function T = TorqueCorrection(H,T,H_max)

if (H_max - abs(H) <= 1e-3)
      T = 0;
else
    T =T;

end

== matlab function Latex/Non Linear SC Dynamics/MATLAB Function1 ==
  data: cubeSatOmega input; q_dot output; q input
function q_dot = omega2qdot(cubeSatOmega,q)

wx = cubeSatOmega(1);
wy = cubeSatOmega(2);
wz = cubeSatOmega(3);

OmegaMatrix = [0 wz -wy wx ;
               -wz 0 wx wy; 
               wy -wx 0 wz;
               -wx -wy -wz 0];
            
q_dot=0.5*OmegaMatrix*q;

end

== matlab function Latex/RWS/RW Simplified7/MATLAB Function ==
  data: H input; T output; T input; H_max input
function T = TorqueCorrection(H,T,H_max)

if (H_max-abs(H) <= 1e-9)
      T = 0;
else
    T =T;

end

== matlab function Latex/RWS/RW Simplified2/MATLAB Function ==
  data: H input; T output; T input; H_max input
function T = TorqueCorrection(H,T,H_max)

if (H_max-abs(H) <= 1e-9)
      T = 0;
else
    T =T;

end

== matlab function Latex/Magnetorquers Model/Corrección X ==
  data: T_error input; B input; T_error output
function T_error = fcn(T_error,B)

if (B(2)> 0)
    HGain =1;
else
    HGain =- 1;

end
T_error = T_error*HGain; 
end

== matlab function Latex/Magnetorquers Model/Corrección Y ==
  data: T_error input; B input; T_error output
function T_error = MgtY_correction(T_error,B)
HGain =1;

if (B(1)>= 0)
    HGain =-1;
else
    HGain =1 ;

end
T_error = T_error*HGain; 
end

== matlab function Latex/Subsystem8/Extract B ==
  data: B_cal input; XYZ_Magnetic output size=[3,1]; time input
function XYZ_Magnetic = fcn(B_cal,time)

index= 1+round(time);
s = size(B_cal);
if index> s(2)
    XYZ_Magnetic = B_cal(:,s(2));
else
    XYZ_Magnetic = B_cal(:,index);
end

== matlab function Latex/Subsystem8/MATLAB Function ==
  data: NEDMagnetic input; RPY_Magnetic output; RPY input
function RPY_Magnetic = RPY_Magnetic(NEDMagnetic,RPY)

R = RPY(1);
P= RPY(2);
Y = RPY(3);



C_NED2ENU = [0 1 0;
             1 0 0
             0 0 -1];
C_RPY2ENU = [sin(Y)*cos(P) cos(R)*cos(Y)+sin(R)*sin(Y)*sin(P) -sin(R)*cos(Y)+cos(R)*sin(Y)*sin(P);
    cos(Y)*cos(P) -cos(R)*sin(Y)+sin(R)*cos(Y)*sin(P) sin(R)*sin(Y)+cos(R)*cos(Y)*sin(P);
    sin(P) -sin(R)*cos(P) -cos(R)*cos(P)];

C_ENU2RPY = C_RPY2ENU^-1; 

RPY_Magnetic = C_ENU2RPY*C_NED2ENU*NEDMagnetic; 


end
